simulink model "relative_test"  (R2022a)
settings: Solver=ode4  StartTime=0.0  StopTime=Simulation_Time  FixedStep=0.1  RelTol=1e-3
values from neighbouring files (symbols this model uses):
  relative_pos0 = [relative_state0(1), relative_state0(2), relative_state0(3)]'    [relative_test_starter.m]
  relative_vel0 = [relative_state0(4), relative_state0(5), relative_state0(6)]'    [relative_test_starter.m]
  SS_Kep_init = [(6371.8 + 550)*km2m 0 45*deg2rad 0*deg2rad 0*deg2rad 0.00002*deg2rad]    [relative_test_starter.m]
  SS_state0 = kepel_statvec(SS_Kep_init)    [relative_test_starter.m]
  TS_Kep_init = [(6371.8 + 550)*km2m 0 45*deg2rad 0*deg2rad 0*deg2rad 0.00000*deg2rad]    [relative_test_starter.m]
  TS_state0 = kepel_statvec(TS_Kep_init)    [relative_test_starter.m]
undefined symbols (not defined in the file or in its folder): X, Y, Z
libraries: nesl_utility x60, sm_lib x27, sharedtransform x1
(part 3 of 3)

== matlab function relative_test/Service SAT vs Target SAT using Kepler/SS Basic Kepler Propagator ==
  data: initial_condition input; dfdt output; State output; eci2lvlh output
function [dfdt, State, eci2lvlh]    = eq_propagate(initial_condition)

u  = 3.9865*10^14;
Re = 6378137; % earth radius in m
sat_mass = 100;%[kg]

dfdt = zeros(size(initial_condition));

x  = initial_condition(1); % x
y  = initial_condition(2); % y
z  = initial_condition(3); % z
x1 = initial_condition(4); % vel_x
y1 = initial_condition(5); % vel_y
z1 = initial_condition(6); % vel_z

r=sqrt(x^2+y^2+z^2);

% % %   Keplar Motion Equatnion
% % %  => r_dd + u/(r^3)r_ = 0 => r_dd = -u/(r^3)r_
dfdt(1) = x1;% vel_x
dfdt(2) = y1;% vel_y
dfdt(3) = z1;% vel_z
% dfdt(4) = -u*x/r^3 + sat_accel(1) + f_vec(1)/sat_mass;% accel_x
% dfdt(5) = -u*y/r^3 + sat_accel(2) + f_vec(2)/sat_mass;% accel_y
% dfdt(6) = -u*z/r^3 + sat_accel(3) + f_vec(3)/sat_mass;% accel_z
dfdt(4) = -u*x/r^3;% accel_x
dfdt(5) = -u*y/r^3;% accel_y
dfdt(6) = -u*z/r^3;% accel_z

State = [x,y,z,x1,y1,z1,dfdt(4),dfdt(5),dfdt(6)]';

% % % % % % % % % % % % LVLH Frame % % % % % % % % % % % % % % % % % % % % % % % % % % % % % % % % % % % %
% x as the unit vector directed along the spacecraft position vector:
lvlh_z = -[x;y;z]./r; 
rcv    = cross([x;y;z],[x1;y1;z1]);
% z as the unit vector directed along the spacecraft's orbital angular momentum vector:
lvlh_y = rcv/norm(rcv);
% y as the unit vector that completes a right handed coordinate system:
lvlh_x = cross(lvlh_z, lvlh_y);

eci2lvlh = [lvlh_x, lvlh_y, lvlh_z];

end

== matlab function relative_test/Service SAT vs Target SAT using Kepler/MATLAB Function ==
  data: ts_state input; rel_pos output; ss_state input; rel_vel output; rel_acc output
function [rel_pos, rel_vel, rel_acc] = fcn(ts_state, ss_state)

ts_pos = [ts_state(1), ts_state(2), ts_state(3)]';
ts_vel = [ts_state(4), ts_state(5), ts_state(6)]';
ts_acc = [ts_state(7), ts_state(8), ts_state(9)]';
ss_pos = [ss_state(1), ss_state(2), ss_state(3)]';
ss_vel = [ss_state(4), ss_state(5), ss_state(6)]';
ss_acc = [ss_state(7), ss_state(8), ss_state(9)]';

rel_pos = ts_pos - ss_pos;
rel_vel = ts_vel - ss_vel;
rel_acc = ts_acc - ss_acc;


end

== matlab function relative_test/SS Basic Kepler Propagator ==
  data: initial_condition input; dfdt output; State output; eci2lvlh output
function [dfdt, State, eci2lvlh]    = eq_propagate(initial_condition)

u  = 3.9865*10^14;
Re = 6378137; % earth radius in m
sat_mass = 100;%[kg]

dfdt = zeros(size(initial_condition));

x  = initial_condition(1); % x
y  = initial_condition(2); % y
z  = initial_condition(3); % z
x1 = initial_condition(4); % vel_x
y1 = initial_condition(5); % vel_y
z1 = initial_condition(6); % vel_z

r=sqrt(x^2+y^2+z^2);

% % %   Keplar Motion Equatnion
% % %  => r_dd + u/(r^3)r_ = 0 => r_dd = -u/(r^3)r_
dfdt(1) = x1;% vel_x
dfdt(2) = y1;% vel_y
dfdt(3) = z1;% vel_z
% dfdt(4) = -u*x/r^3 + sat_accel(1) + f_vec(1)/sat_mass;% accel_x
% dfdt(5) = -u*y/r^3 + sat_accel(2) + f_vec(2)/sat_mass;% accel_y
% dfdt(6) = -u*z/r^3 + sat_accel(3) + f_vec(3)/sat_mass;% accel_z
dfdt(4) = -u*x/r^3;% accel_x
dfdt(5) = -u*y/r^3;% accel_y
dfdt(6) = -u*z/r^3;% accel_z

State = [x,y,z,x1,y1,z1,dfdt(4),dfdt(5),dfdt(6)]';

% % % % % % % % % % % % LVLH Frame % % % % % % % % % % % % % % % % % % % % % % % % % % % % % % % % % % % %
% x as the unit vector directed along the spacecraft position vector:
lvlh_z = -[x;y;z]./r; 
rcv    = cross([x;y;z],[x1;y1;z1]);
% z as the unit vector directed along the spacecraft's orbital angular momentum vector:
lvlh_y = rcv/norm(rcv);
% y as the unit vector that completes a right handed coordinate system:
lvlh_x = cross(lvlh_z, lvlh_y);

eci2lvlh = [lvlh_x, lvlh_y, lvlh_z];

end

== matlab function relative_test/TS Basic Kepler Propagator ==
  data: initial_condition input; dfdt output; State output; eci2lvlh output
function [dfdt, State, eci2lvlh]    = eq_propagate(initial_condition)

u  = 3.9865*10^14;
Re = 6378137; % earth radius in m
sat_mass = 100;%[kg]

dfdt = zeros(size(initial_condition));

x  = initial_condition(1); % x
y  = initial_condition(2); % y
z  = initial_condition(3); % z
x1 = initial_condition(4); % vel_x
y1 = initial_condition(5); % vel_y
z1 = initial_condition(6); % vel_z

r=sqrt(x^2+y^2+z^2);

% % %   Keplar Motion Equatnion
% % %  => r_dd + u/(r^3)r_ = 0 => r_dd = -u/(r^3)r_
dfdt(1) = x1;% vel_x
dfdt(2) = y1;% vel_y
dfdt(3) = z1;% vel_z
% dfdt(4) = -u*x/r^3 + sat_accel(1) + f_vec(1)/sat_mass;% accel_x
% dfdt(5) = -u*y/r^3 + sat_accel(2) + f_vec(2)/sat_mass;% accel_y
% dfdt(6) = -u*z/r^3 + sat_accel(3) + f_vec(3)/sat_mass;% accel_z
dfdt(4) = -u*x/r^3;% accel_x
dfdt(5) = -u*y/r^3;% accel_y
dfdt(6) = -u*z/r^3;% accel_z

State = [x,y,z,x1,y1,z1,dfdt(4),dfdt(5),dfdt(6)]';

% % % % % % % % % % % % LVLH Frame % % % % % % % % % % % % % % % % % % % % % % % % % % % % % % % % % % % %
% x as the unit vector directed along the spacecraft position vector:
lvlh_z = -[x;y;z]./r; 
rcv    = cross([x;y;z],[x1;y1;z1]);
% z as the unit vector directed along the spacecraft's orbital angular momentum vector:
lvlh_y = rcv/norm(rcv);
% y as the unit vector that completes a right handed coordinate system:
lvlh_x = cross(lvlh_z, lvlh_y);

eci2lvlh = [lvlh_x, lvlh_y, lvlh_z];

end

== matlab function relative_test/MATLAB Function2 ==
  data: statv input; kepel output
function kepel  = statvec_kepel (statv)
% [kepel] = statvec_kepel (statv)
%
%	The function statvec_kepel transforms the state vector statv
%	into the corresponding keplerian elements in the
%	same reference system.
%
% Input:
%	statv
%		state vector in meters and meters/second.
%
% Output:
%	statvec_kepel
%		vector containing the keplerian elements:
%		(1) - semimajor axis of the orbit in meters.
%		(2) - eccentricity.
%		(3) - inclination in radians.
%		(4) - right ascension of ascending node in radians.
%		(5) - argument of perigee in radians.
%		(6) - mean anomaly in radians.
%
% Authors:
%	Helio K. Kuga
%    Valder M. Medeiros
%	Valdemir Carrara			february/80			version 1.0
%	Helio K. Kuga     			august/82           version 2.0
%	Ulisses T V Guedes 			december/95	 		version 2.1
%               - fix perigee procedure when orbit plane
%                  equal to equatorial plane
%	Valdemir Carrara 			july/05				(C version)
%   Valdemir Carrara            March/09        Matlab

EARTH_GRAVITY	= 3.9860064e+14;		% Earth's gravitational constant (m**3/s**2)

xp  = [statv(1) statv(2) statv(3)];
xv  = [statv(4) statv(5) statv(6)];
r      = sqrt(xp*xp');
vq     = xv*xv';
ainv   = 2.0/r - vq/EARTH_GRAVITY;

h      = cross(xp, xv);
hm     = sqrt(h*h');
an = [0 0 0];
if (hm < 1.e-10)
    disp (' *** Message from function statvec_kepel: *** ');
    disp (' There are no keplerian elements corresponding to this state vector');
    kepel = [0, 0, 0, 0, 0, 0];
else
    h      = h/hm;
    incl   = acos(h(3));
    raan   = atan2(h(1), -h(2));
    d      = xp*xv' / EARTH_GRAVITY;
    esene  = d * sqrt(EARTH_GRAVITY*ainv);
    ecose  = 1 - r*ainv;
    exc    = sqrt(esene*esene + ecose*ecose);
    E      = atan2(esene, ecose);
    mean   = mod (E - esene, 2*pi);
    if mean < 0
        mean = mean + 2*pi;
    end

    if exc < 1.e-10
        arpe = 0;
    else
        dp     = 1./r - ainv;
        ev     = dp*xp - d*xv;
        abev   = sqrt(ev*ev');
        ev     = ev/abev;
        an(1)  = cos(raan);
        an(2)  = sin(raan);
        an(3)  = 0;
        fi     = ev*cross(h, an)';
        arpe = acos(ev*an');
        if fi < 0
            arpe  =  -arpe + 2*pi;
        end
    end

    kepel = [1./ainv, exc, incl, raan, arpe, mean];
end

end

== matlab function relative_test/MATLAB Function3 ==
  data: kepler input; ra output; rp output; T output; T_hour output; we output
function [ra, rp, T, T_hour, we] = fcn(kepler)

u=3.9865*10^14;

a = kepler(1);
e = kepler(2);
% 

ra = a*(1+e);%장반경
rp = a*(1-e);%단반경

a = (ra+rp)/2;% semi-major axis

% a = (550 + 6371.8)*1000;

T = 2*pi*sqrt((a*a*a)/(u));

T_hour = T/3600;

we = 2*pi/T;
% we = 1.1207*0.001;

end

== matlab function relative_test/MATLAB Function4 ==
  data: q input; cntl_out output; w input
function cntl_out = LVLH_Attitude_Control(q, w)

qs = q(1);
qv = [q(2), q(3), q(4)]';
w  = [w(1), w(2), w(3)]';

K1 = diag([0.05 0.05 0.05]);
K2 = diag([0.4 0.4 0.4]);

cntl_out = K1*qv - K2*w;

end

== matlab function relative_test/Service SAT vs Target SAT using Kepler/TS Basic Kepler Propagator ==
  data: initial_condition input; dfdt output; State output; eci2lvlh output
function [dfdt, State, eci2lvlh]    = eq_propagate(initial_condition)

u  = 3.9865*10^14;
Re = 6378137; % earth radius in m
sat_mass = 100;%[kg]

dfdt = zeros(size(initial_condition));

x  = initial_condition(1); % x
y  = initial_condition(2); % y
z  = initial_condition(3); % z
x1 = initial_condition(4); % vel_x
y1 = initial_condition(5); % vel_y
z1 = initial_condition(6); % vel_z

r=sqrt(x^2+y^2+z^2);

% % %   Keplar Motion Equatnion
% % %  => r_dd + u/(r^3)r_ = 0 => r_dd = -u/(r^3)r_
dfdt(1) = x1;% vel_x
dfdt(2) = y1;% vel_y
dfdt(3) = z1;% vel_z
% dfdt(4) = -u*x/r^3 + sat_accel(1) + f_vec(1)/sat_mass;% accel_x
% dfdt(5) = -u*y/r^3 + sat_accel(2) + f_vec(2)/sat_mass;% accel_y
% dfdt(6) = -u*z/r^3 + sat_accel(3) + f_vec(3)/sat_mass;% accel_z
dfdt(4) = -u*x/r^3;% accel_x
dfdt(5) = -u*y/r^3;% accel_y
dfdt(6) = -u*z/r^3;% accel_z

State = [x,y,z,x1,y1,z1,dfdt(4),dfdt(5),dfdt(6)]';

% % % % % % % % % % % % LVLH Frame % % % % % % % % % % % % % % % % % % % % % % % % % % % % % % % % % % % %
% x as the unit vector directed along the spacecraft position vector:
lvlh_z = -[x;y;z]./r; 
rcv    = cross([x;y;z],[x1;y1;z1]);
% z as the unit vector directed along the spacecraft's orbital angular momentum vector:
lvlh_y = rcv/norm(rcv);
% y as the unit vector that completes a right handed coordinate system:
lvlh_x = cross(lvlh_z, lvlh_y);

eci2lvlh = [lvlh_x, lvlh_y, lvlh_z];

end
